simulink model "GFo_L_Filter"  (R2016a)
settings: Solver=ode1  SolverMode=SingleTasking  StartTime=0.0  StopTime=4  FixedStep=Time_Step  MaxStep=1e-4  RelTol=1e-3
PreLoadFcn:
  | GFo_L_Filter_Init;
InitFcn:
  | GFo_L_Filter_Init;
undefined symbols (not defined in the file): GRD00_Lg, GRD00_Rg, Time_Step
libraries: powerlib x7, Source_Lib x1, GFo_Lib x1
settings Model: Creator=Frederic_Colas  LastModifiedBy=fcolas
settings DebuggingCC: UnconnectedInputMsg=none  UnconnectedOutputMsg=none  UnconnectedLineMsg=none  SFUnexpectedBacktrackingDiag=error  SFNoUnconditionalDefaultTransitionDiag=error
settings HardwareCC: ProdWordSize=32  ProdHWDeviceType=Specified
settings GRTTargetCC: TargetLangStandard=C99 (ISO)
settings ConfigComp: CovMetricSettings=dwe  CovSaveCumulativeToWorkspaceVar=off  CovSaveSingleToWorkspaceVar=off  CovExternalEMLEnable=on
settings SimscapeCC: SimscapeNormalizeSystem=off

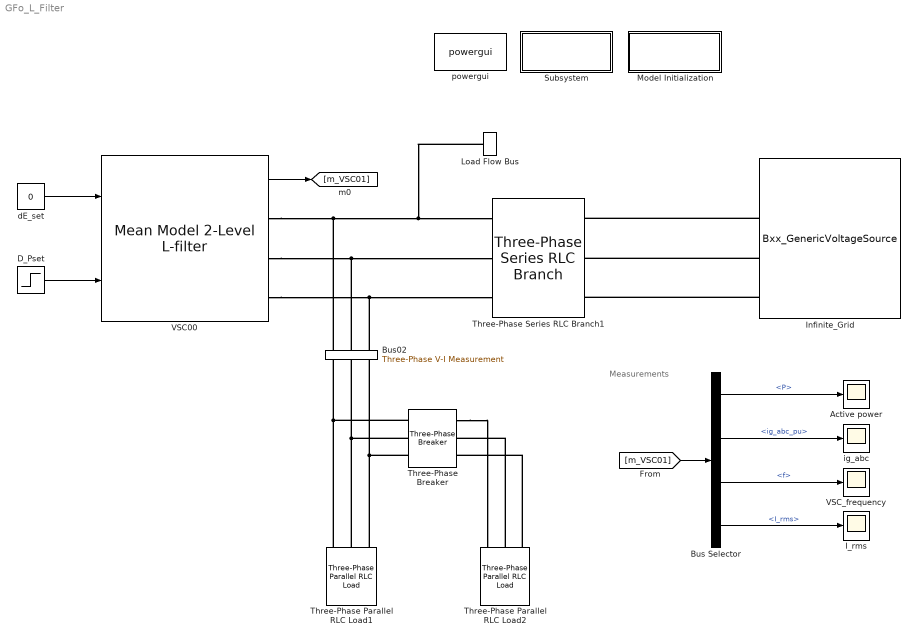
== system GFo_L_Filter ==
  note: Measurements
  Active power : Scope
  Bus Selector : BusSelector  OutputSignals=P,I.ig_abc_pu,f,VI.I_rms
  "Bus02 " : powerlib/Measurements/Three-Phase V-I Measurement  VoltageMeasurement=no  SetLabelV=off  LabelV=Vabc  Vpu=off  VpuLL=off  CurrentMeasurement=no  SetLabelI=off  LabelI=Iabc  Ipu=off  Pbase=100e6  Vbase=500e3  OutputType=Complex  PhasorSimulation=off  PSBequivalent=0
  D_Pset : Step  After=0.68  SampleTime=0
  I_rms : Scope
  Infinite_Grid : Source_Lib/Bxx_GenericVoltageSource  SourceNature_str=INFINITE  fn=50  Sn=1000e6  Un=Ug  LFpopup=Swing  P0=-199451393.8731  Q0=1988404.547  V0_pu=1  U0=20000  Theta0_deg=0  H_s=5  DroopOnOff=on  R_percent=4  TN=1  TD=2
  Load Flow Bus : powerlib/Measurements/Load Flow Bus  LConnTagsString=a  Phases=single  Connectors=on one side  ID=BUS_1  Vbase=Ug  Vref=1  Vangle=0  VLF=1.001  VLFb=1  VLFc=1  angleLF=0.5714  angleLFb=0  angleLFc=0
  Model Initialization : Subsystem  mask(Model Functions){InitFcnX=GFo_L_Filter_Init;, prel=on, posl=off, inif=on, strf=off}
      mask prompts: InitFcnX "Initialisation"; prel "Preload Function"; posl "PostLoad Function"; inif "InitFcn"; strf "StartFcn"
      mask init:
      | currentBlock = gcb;
      | root = bdroot(currentBlock);
      | 
      | if ~strcmp(get_param(root,'BlockDiagramType'),'library')
      |     if prel==1
      |         set_param(root, 'PreLoadFcn', InitFcnX);
      |     else
      |         set_param(root, 'PreLoadFcn', '');
      |     end
      |     if inif==1
      |         set_param(root, 'InitFcn', InitFcnX);
      |     else
      |         set_param(root, 'InitFcn', '');
      |     end
      |     if strf==1
      |         set_param(root, 'StartFcn', InitFcnX);
      |     else
      |         set_param(root, 'StartFcn', '');
      |     end
      |     if posl==1
      |         set_param(root, 'PostLoadFcn', InitFcnX);
      |     else
      |         set_param(root, 'PostLoadFcn', '');
      |     end
      | end
      | 
      | pos = get_param(currentBlock, 'Position');
      | width = pos(3) - pos(1); height = pos(4) - pos(2);
      | txt = [ upper(root) '\n' '- InitFcn. . . . . '  get_param(root, 'InitFcn') ];
      settings: CopyFcn=set_param(gcb,'LinkStatus','none')
      mask Display:
      | %text(5, height*0.5, txt, 'horizontalAlignment', 'left', 'verticalAlignment', 'middle') ;
      | color('blue'),disp('Initialization Function\nParameters')
  Subsystem : Subsystem
      settings: OpenFcn=LoadFlow_VSC
      mask Display: color('blue'),disp('Update Loadflow')
  Three-Phase Parallel RLC Load1 : powerlib/Elements/Three-Phase Parallel RLC Load  LConnTagsString=A|B|C  Configuration=Y (grounded)  NominalVoltage=Ug  Vabc=[1e3 1e3 1e3]  Vabcp=[1e3 1e3 1e3]  NominalFrequency=fb  UnbalancedPower=off  ActivePower=100e6  InductivePower=0  CapacitivePower=0  Pabc=[10e3 9e3 11e3]  QLabc=[100 90 110]  QCabc=[100 90 110]  Pabcp=[10e3 9e3 11e3]  QLabcp=[100 90 110]  QCabcp=[100 90 110]  Measurements=None  LoadType=constant Z
  Three-Phase Parallel RLC Load2 : powerlib/Elements/Three-Phase Parallel RLC Load  LConnTagsString=A|B|C  Configuration=Y (grounded)  NominalVoltage=Ug  Vabc=[1e3 1e3 1e3]  Vabcp=[1e3 1e3 1e3]  NominalFrequency=fb  UnbalancedPower=off  ActivePower=1000e6  InductivePower=0  CapacitivePower=0  Pabc=[10e3 9e3 11e3]  QLabc=[100 90 110]  QCabc=[100 90 110]  Pabcp=[10e3 9e3 11e3]  QLabcp=[100 90 110]  QCabcp=[100 90 110]  Measurements=None  LoadType=constant Z
  Three-Phase Series RLC Branch1 : powerlib/Elements/Three-Phase Series RLC Branch  LConnTagsString=A|B|C  RConnTagsString=A|B|C  BranchType=RL  Resistance=GRD00_Rg  Inductance=GRD00_Lg  Capacitance=1e-6  Measurements=None
  Three-Phase Breaker : powerlib/Elements/Three-Phase Breaker  InitialState=open  SwitchA=on  SwitchB=on  SwitchC=on  SwitchTimes=2  External=off  BreakerResistance=0.01  SnubberResistance=1e6  SnubberCapacitance=inf  Measurements=None
  VSC00 : GFo_Lib/Mean Model 2-Level L-filter  fn=50  Sn=1000e6  Pn=1000e6  Udcn=640e3  Time_Step=Time_Step  Un1=320e3  Un2=Ug  Rt_pu=0.005  Lt_pu=0.15  Lm_pu=500  Rm_pu=500  Tr_PLL=10  Val_Freq_Support=on  R_percent=4  Rv=0.09  W_TVR=60  I_thresh_pu=1.2  DX_DR=5  Kp_Rvi_pu=0.676  I_max_pu=1.2  Tr_I_max=10  Advanced=on  gainpopup=Inertia Less  f_Inertia_Less=5/(2*pi)  zeta_Inertia_Less=1  Param_Inertia=PI  H_GFo=5  zeta_GFo=0.7  LFpopup=PQ  P0=0.3  Q0=2.3716e-08  V0=1.0009  Theta0=0.57142
  VSC_frequency : Scope
  dE_set : Constant  Value=0
  ig_abc : Scope
  powergui : powerlib/powergui  Priority=1  SimulationMode=Discrete  SampleTime=Time_Step  frequency=60  Iterations=50  frequencyindice=50  Pbase=1000000000  ErrMax=1e-6  UnitsV=kV  UnitsW=MW  buscounter=0  FunctionMessages=off  echomessages=off  EnableUseOfTLC=off  CurrentSourceSwitches=off  DisableSnubberDevices=off  DisableRonSwitches=off  DisableVfSwitches=off  DisplayEquations=off  AutomaticDiscreteSolvers=off  SolverType=Tustin/Backward Euler (TBE)  Interpol=off  ExternalGateDelay=off  methode=off  Ts=100  x0status=blocks  SPID=on  SwTol=0  HookPort=off  NonlinearTolerance=1e-4  nMaxIteration=100  ContinueOnMaxIteration=off  RestoreLinks=warning  ResistiveCurrentMeasurement=off  Frange=[0:2:500]  Ylog=off  Xlog=on  ShowGrid=off  save=off  variable=ZData  structure=0  ZoomFFT=off  StartTime=0.0  cycles=1  DisplayStyle=1  fundamental=60  FreqAxis=off  MaxFrequency=1000  frequencyindicesteady=1  RmsSteady=1  display=off
  wires:
  dE_set/1 -> VSC00/1
  D_Pset/1 -> VSC00/2
  [m_VSC01] -> Bus Selector/1
  Bus Selector/1 -> Active power/1  "<P>"
  VSC00/1 -> [m_VSC01]
  Bus Selector/2 -> ig_abc/1  "<ig_abc_pu>"
  Bus Selector/3 -> VSC_frequency/1  "<f>"
  Bus Selector/4 -> I_rms/1  "<I_rms>"
  connections:
  VSC00/RConn1 -- "Bus02 "/LConn3 -- Load Flow Bus/LConn1 -- Three-Phase Series RLC Branch1/LConn1
  VSC00/RConn3 -- "Bus02 "/LConn1 -- Three-Phase Series RLC Branch1/LConn3
  VSC00/RConn2 -- "Bus02 "/LConn2 -- Three-Phase Series RLC Branch1/LConn2
  Infinite_Grid/RConn1 -- Three-Phase Series RLC Branch1/RConn1
  Infinite_Grid/RConn2 -- Three-Phase Series RLC Branch1/RConn2
  Infinite_Grid/RConn3 -- Three-Phase Series RLC Branch1/RConn3
  Three-Phase Parallel RLC Load1/LConn2 -- "Bus02 "/RConn2 -- Three-Phase Breaker/LConn2
  Three-Phase Parallel RLC Load1/LConn3 -- "Bus02 "/RConn1 -- Three-Phase Breaker/LConn3
  Three-Phase Parallel RLC Load1/LConn1 -- "Bus02 "/RConn3 -- Three-Phase Breaker/LConn1
  Three-Phase Parallel RLC Load2/LConn3 -- Three-Phase Breaker/RConn3
  Three-Phase Parallel RLC Load2/LConn2 -- Three-Phase Breaker/RConn2
  Three-Phase Breaker/RConn1 -- Three-Phase Parallel RLC Load2/LConn1

== system GFo_L_Filter/Model Initialization ==

== system GFo_L_Filter/Subsystem ==
